simulink model "Subsystem0"  (R2020b)
settings: Solver=VariableStepAuto  StartTime=0.0  StopTime=10.0  RelTol=1e-3
settings Model: Creator=hp  LastModifiedBy=hp
settings DataIOCC: SaveOutput=off  SaveTime=off

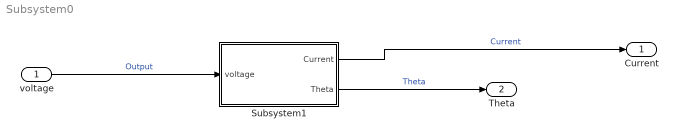
== system Subsystem0 ==
  voltage : Inport  OutDataTypeStr=double  PortDimensions=1  SampleTime=0
  Subsystem1 : Subsystem
  Current : Outport  OutDataTypeStr=double  PortDimensions=1  SampleTime=0
  Theta : Outport  Port=2  OutDataTypeStr=double  PortDimensions=1  SampleTime=0
  wires:
  Subsystem1/2(Theta) -> Theta/1  "Theta"
  voltage/1 -> Subsystem1/1(voltage)  "Output"
  Subsystem1/1(Current) -> Current/1  "Current"

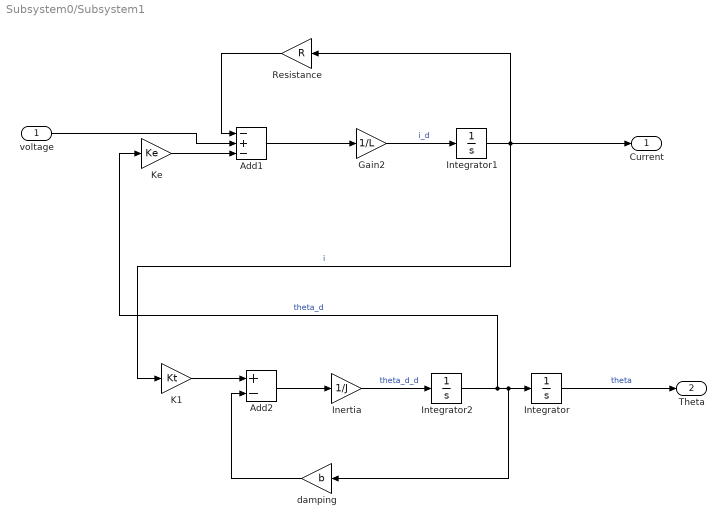
== system Subsystem0/Subsystem1 ==
  voltage : Inport
  Add1 : Sum  Inputs=-+-
  Add2 : Sum  Inputs=+-
  Gain2 : Gain  Gain=1/L  mask{L=2.75*10^(-6)}
  Inertia : Gain  Gain=1/J  mask{J=3.2284*10^(-6)}
  Integrator : Integrator
  Integrator1 : Integrator
  Integrator2 : Integrator
  K1 : Gain  Gain=Kt  mask{Kt=0.0274}
  Ke : Gain  Gain=Ke  mask{Ke=0.0274}
  Resistance : Gain  Gain=R  mask{R=4}
  damping : Gain  Gain=b  mask{b=3.5077*10^(-6)}
  Current : Outport
  Theta : Outport  Port=2
  wires:
  K1/1 -> Add2/1
  Resistance/1 -> Add1/1
  Gain2/1 -> Integrator1/1  "i_d"
  Add2/1 -> Inertia/1
  damping/1 -> Add2/2
  Integrator2/1 -> Ke/1, damping/1, Integrator/1  "theta_d"
  Ke/1 -> Add1/3
  Inertia/1 -> Integrator2/1  "theta_d_d"
  Add1/1 -> Gain2/1
  voltage/1 -> Add1/2
  Integrator1/1 -> Resistance/1, K1/1, Current/1  "i"
  Integrator/1 -> Theta/1  "theta"
